simulink model "NelinModel"  (R2020b)
settings: Solver=VariableStepAuto  StartTime=0.0  StopTime=10.0  RelTol=1e-3
undefined symbols (not defined in the file): g, L
settings Model: Creator=kpass  LastModifiedBy=kpass

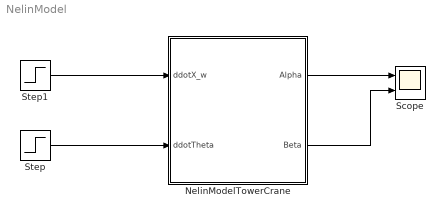
== system NelinModel ==
  NelinModelTowerCrane : Subsystem
  Scope : Scope  NumInputPorts=2
  Step : Step  Time=2  SampleTime=0
  Step1 : Step  After=2  SampleTime=0
  wires:
  NelinModelTowerCrane/1(Alpha) -> Scope/1
  NelinModelTowerCrane/2(Beta) -> Scope/2
  Step/1 -> NelinModelTowerCrane/2(ddotTheta)
  Step1/1 -> NelinModelTowerCrane/1(ddotX_w)

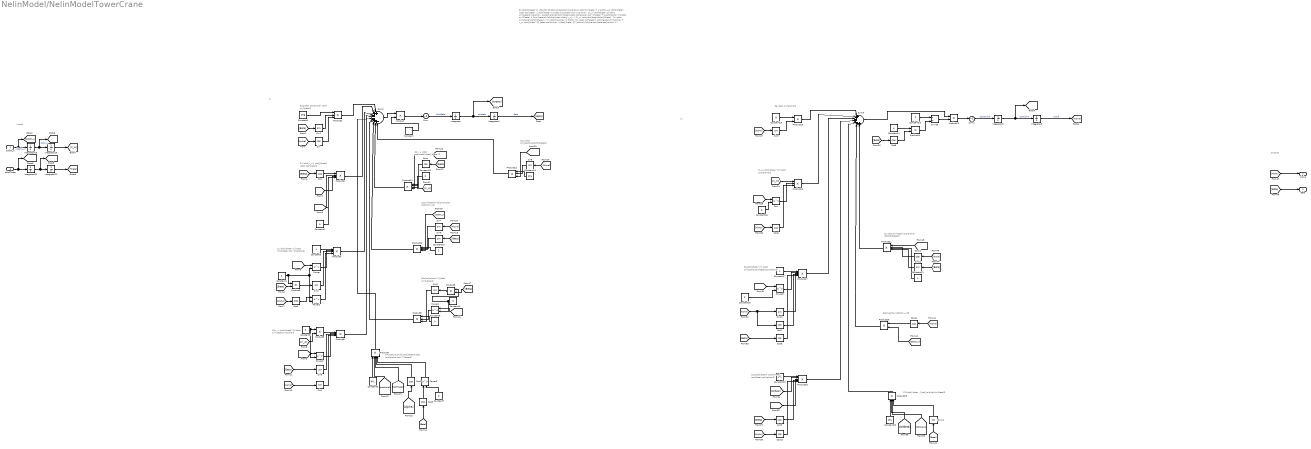
== system NelinModel/NelinModelTowerCrane ==
  note: Outputs
  note: 2)
  note: $L \cdot sin(\beta) cos(\alpha) \ddot{\theta}$
  note: $cos(\alpha) \ddot{x_w}$
  note: $2L\dot{\beta}\dot{\alpha}sin(\beta)$
  note: $2L\dot{\beta} \dot{\theta} cos(\beta) cos(\alpha)$
  note: $L\dot{\theta^2} \cdot sin(\alpha)cos(\beta)cos(\alpha)$
  note: $x_w \dot{\theta^2} \cdot cos(\alpha)$
  note: $g \cdot sin(\alpha)$
  note: Inputs
  note: 1)
  note: $2L \cdot sin(\alpha)\ddot{\theta}$
  note: $2x_w \cdot cos(\beta)\ddot{\theta}$
  note: $2sin(\beta)sin(\alpha)\cdot \ddot{x}_w$
  note: $L\dot{\alpha^2}\cdot sin(2\beta)$
  note: $4L\dot{\alpha}\dot{\theta}\cdot cos(\alpha) cos^2(\beta)$
  note: $2x_w \dot{\theta^2}\cdot sin(\beta)sin(\alpha)$
  note: $L \dot{\theta^2}\cdot sin(2\beta) cos^2(\alpha)$
  note: $4 \dot{x_w} \dot{\theta} \cdot cos(\beta)$
  note: $2g\cdot cos(\alpha) \cdot sin(\beta)$
  note: $1)\ddot{\beta} = -\frac{1}{2\cdot L}(2g\cdot cos(\alpha) \cdot sin(\beta) + 4 \dot{x_w} \dot{\theta} \cdot cos(\beta) - L \dot{\theta^2}\cdot sin(2\beta) cos^2(\alpha) - 2x_w \dot{\theta^2}\cdot sin(\beta)sin(\alpha) - 4L\dot{\alpha}\dot{\theta}\cdot cos(\alpha) cos^2(\beta) + L\dot{\alpha^2}\cdot sin(2\beta) + 2sin(\beta)sin(\alpha)\cdot \ddot{x_w} + 2x_w \cdot cos(\beta)\ddot{\theta} - 2L \cdot sin(\alpha)\ddot{\theta}) \\ 2) \ddot{\alpha} = \frac{1}{L \cdot cos(\beta)} \cdot (g\cdot sin(\alpha) + x_w \dot{\theta^2} \cdot cos(\alpha) - L\dot{\theta^2} \cdot sin(\alpha)cos(\beta)cos(\alpha) + 2L\dot{\beta} \dot{\theta} cos(\beta) cos(\alpha) - 2L\dot{\beta}\dot{\alpha}sin(\beta) - cos(\alpha) \ddot{x_w} + L \cdot sin(\beta) cos(\alpha) \ddot{\theta})$
  ddotX_w : Inport
  ddotTheta : Inport  Port=2
  Constant : Constant  Value=1/(2*L)
  Constant1 : Constant  Value=2*g
  Constant{4..5,7,9..11,16,18} (8 alike) : Constant  Value=2
  Constant12 : Constant  Value=2*L
  Constant13 : Constant
  Constant{3,8,14,17,21} (5 alike) : Constant  Value=L
  Constant15 : Constant  Value=g
  Constant19 : Constant  Value=2*L
  Constant2 : Constant  Value=4
  Constant20 : Constant  Value=2*L
  Constant6 : Constant  Value=4*L
  Cos{,1..12} (13 alike) : Trigonometry  Operator=cos
  Divide : Product  Inputs=*/
  Integrator{,1..3,18,20..21} (7 alike) : Integrator
  Integrator19 : Integrator  InitialCondition=1
  Pow : Math  Operator=pow  RndMeth=Zero  SaturateOnIntegerOverflow=on
  Power{,1..5} (6 alike) : Math  Operator=pow  SaturateOnIntegerOverflow=on
  Product{,3,5,8,13..15,20} (8 alike) : Product
  Product{1,9,12,16} (4 alike) : Product  Inputs=3
  Product{2,4,6,10..11,19,21} (7 alike) : Product  Inputs=4
  Product17 : Product  Inputs=5
  Product18 : Product  Inputs=5
  Product7 : Product  Inputs=5
  Sin : Trigonometry  Operator=cos
  Sin{1..12} (12 alike) : Trigonometry
  Sum : Sum  Inputs=-
  Sum1 : Sum  Inputs=-
  Sum2 : Sum  Inputs=|++---+++-
  Sum3 : Sum  Inputs=|++-+--+
  Alpha : Outport
  Beta : Outport  Port=2
  wires:
  Sin/1 -> Product1/3
  Constant1/1 -> Product1/1
  Integrator1/1 -> [Beta]  "Beta"
  Sin1/1 -> Product1/2
  Integrator3/1 -> [Alpha]  "Alpha"
  Sum/1 -> Integrator/1  "ddotBeta"
  Integrator2/1 -> [dotAlpha], Integrator3/1  "dotAlpha"
  Product1/1 -> Sum2/1
  Integrator/1 -> [dotBeta], Integrator1/1  "dotBeta"
  Sum1/1 -> Integrator2/1  "ddotAlpha"
  Constant/1 -> Product/2
  Sum2/1 -> Product/1
  Product/1 -> Sum/1
  [Beta] -> Sin1/1
  [Alpha] -> Sin/1
  [Beta] -> Cos/1
  Cos/1 -> Product2/1
  [dotX_w] -> Product2/3
  [dotTheta] -> Product2/2
  Constant2/1 -> Product2/4
  Product2/1 -> Sum2/2
  [dotTheta] -> Power/1
  Constant4/1 -> Power1/2, Power/2, Product3/1
  [Beta] -> Product3/2
  Product3/1 -> Sin2/1
  [Alpha] -> Cos1/1
  Cos1/1 -> Power1/1
  Constant3/1 -> Product4/1
  Power/1 -> Product4/2
  Sin2/1 -> Product4/3
  Power1/1 -> Product4/4
  Product4/1 -> Sum2/3
  Constant5/1 -> Product5/1, Power2/2
  [X_w] -> Product5/2
  [dotTheta] -> Power2/1
  [Beta] -> Sin3/1
  [Alpha] -> Sin4/1
  Product5/1 -> Product6/1
  Power2/1 -> Product6/2
  Sin3/1 -> Product6/3
  Sin4/1 -> Product6/4
  Product6/1 -> Sum2/4
  Constant7/1 -> Power3/2
  Cos3/1 -> Power3/1
  [Beta] -> Cos3/1
  [Alpha] -> Cos2/1
  Constant6/1 -> Product7/1
  [dotAlpha] -> Product7/2
  [dotTheta] -> Product7/3
  Cos2/1 -> Product7/4
  Power3/1 -> Product7/5
  Product7/1 -> Sum2/5
  [dotAlpha] -> Power4/1
  Constant9/1 -> Product8/1, Power4/2
  [Beta] -> Product8/2
  Product8/1 -> Sin5/1
  Constant8/1 -> Product9/1
  Power4/1 -> Product9/2
  Sin5/1 -> Product9/3
  Product9/1 -> Sum2/6
  Constant10/1 -> Product10/1
  Sin6/1 -> Product10/2
  Sin7/1 -> Product10/3
  [ddotX_w] -> Product10/4
  [Beta] -> Sin6/1
  [Alpha] -> Sin7/1
  Product10/1 -> Sum2/7
  [Beta] -> Cos4/1
  [X_w] -> Product11/1
  Constant11/1 -> Product11/2
  Cos4/1 -> Product11/3
  [ddotTheta] -> Product11/4
  Product11/1 -> Sum2/8
  [Alpha] -> Sin8/1
  Constant12/1 -> Product12/1
  Sin8/1 -> Product12/2
  [ddotTheta] -> Product12/3
  Product12/1 -> Sum2/9
  Product13/1 -> Sum1/1
  Divide/1 -> Product13/2
  Constant13/1 -> Divide/1
  Product14/1 -> Divide/2
  Constant14/1 -> Product14/1
  Cos5/1 -> Product14/2
  [Beta] -> Cos5/1
  Sum3/1 -> Product13/1
  [Alpha] -> Sin9/1
  Constant15/1 -> Product15/1
  Sin9/1 -> Product15/2
  Product15/1 -> Sum3/1
  [dotTheta] -> Pow/1
  Constant16/1 -> Pow/2
  [Alpha] -> Cos6/1
  [X_w] -> Product16/1
  Pow/1 -> Product16/2
  Cos6/1 -> Product16/3
  Product16/1 -> Sum3/2
  [dotTheta] -> Power5/1
  Constant18/1 -> Power5/2
  [Alpha] -> Cos7/1, Sin10/1
  [Beta] -> Cos8/1
  Constant17/1 -> Product17/1
  Power5/1 -> Product17/2
  Sin10/1 -> Product17/3
  Cos7/1 -> Product17/4
  Cos8/1 -> Product17/5
  Product17/1 -> Sum3/3
  [Beta] -> Cos9/1
  [Alpha] -> Cos10/1
  Constant19/1 -> Product18/1
  [dotBeta] -> Product18/2
  [dotTheta] -> Product18/3
  Cos9/1 -> Product18/4
  Cos10/1 -> Product18/5
  Product18/1 -> Sum3/4
  [Beta] -> Sin11/1
  Constant20/1 -> Product19/1
  [dotBeta] -> Product19/2
  [dotAlpha] -> Product19/3
  Sin11/1 -> Product19/4
  Product19/1 -> Sum3/5
  [Alpha] -> Cos11/1
  Cos11/1 -> Product20/1
  [ddotX_w] -> Product20/2
  Product20/1 -> Sum3/6
  [Beta] -> Sin12/1
  [Alpha] -> Cos12/1
  [ddotTheta] -> Product21/1
  Cos12/1 -> Product21/2
  Sin12/1 -> Product21/4
  Constant21/1 -> Product21/3
  Product21/1 -> Sum3/7
  [Alpha] -> Alpha/1
  [Beta] -> Beta/1
  ddotX_w/1 -> Integrator18/1, [ddotX_w]  "ddotX_w"
  Integrator18/1 -> [dotX_w], Integrator19/1  "dotX_w"
  Integrator19/1 -> [X_w]
  ddotTheta/1 -> [ddotTheta], Integrator20/1
  Integrator20/1 -> [dotTheta], Integrator21/1
  Integrator21/1 -> [Theta]
